simulink model "controladorLEAD"  (R2024b)
settings: Solver=VariableStepAuto  StartTime=0.0  StopTime=50  RelTol=1e-3
values from neighbouring files (symbols this model uses):
  planta = obterPlanta()    [obterMalhaAngular.m]    (also in obterMalhaTangencial.m; simularBarra.m; simularRampa.m)
  saturacoes = obterSaturacao()    [simularBarra.m]    (also in simularRampa.m = obterValoresSaturacao())
  x0 = [Mp_req, t_req]    [ajustarRequisitosEstabilidade.m]
undefined symbols (not defined in the file or in its folder): controlador, theta0
libraries: simulink x1
settings Model: Creator=josal  LastModifiedBy=quantks

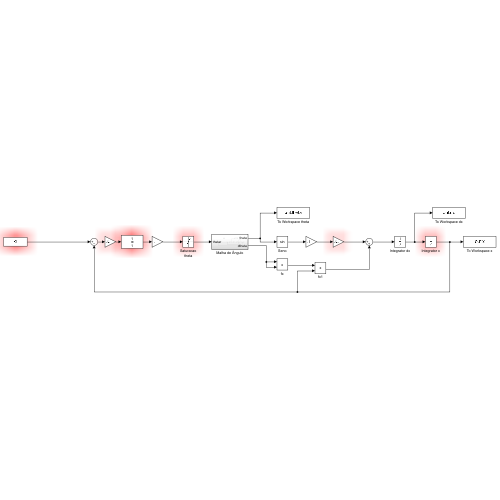
[thumbnail: Simulink's stored preview of the top-level diagram]
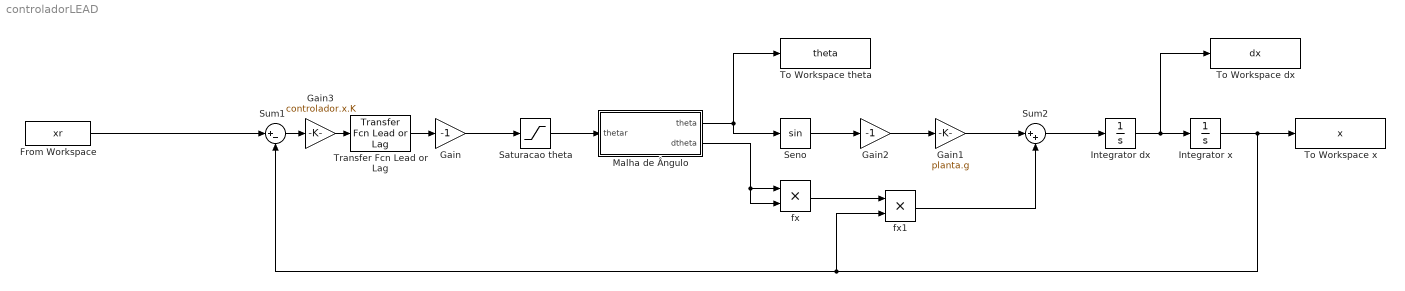
== system controladorLEAD ==
  From Workspace : FromWorkspace  VariableName=xr
  Gain : Gain  Gain=-1
  Gain1 : Gain  Gain=planta.g
  Gain2 : Gain  Gain=-1
  Gain3 : Gain  Gain=controlador.x.K
  Integrator dx : Integrator
  Integrator x : Integrator  InitialCondition=x0
  Malha de Ângulo : Subsystem
  Saturacao theta : Saturate  UpperLimit=saturacoes.sat_theta  LowerLimit=-saturacoes.sat_theta
  Seno : Trigonometry
  Sum1 : Sum  Inputs=|+-
  Sum2 : Sum  Inputs=|++
  To Workspace dx : ToWorkspace  VariableName=dx  SaveFormat=Structure With Time  SampleTime=-1
  To Workspace theta : ToWorkspace  VariableName=theta  SaveFormat=Structure With Time  SampleTime=-1
  To Workspace x : ToWorkspace  VariableName=x  SaveFormat=Structure With Time  SampleTime=-1
  Transfer Fcn Lead or Lag : simulink/Discrete/Transfer Fcn Lead or Lag  PoleZ=-1/(controlador.x.alpha*controlador.x.T)  ZeroZ=-1/(controlador.x.T)  ICPrevOutput=0.0  ICPrevInput=0.0  DoSatur=off
  fx : Product
  fx1 : Product
  wires:
  From Workspace/1 -> Sum1/1
  Integrator dx/1 -> To Workspace dx/1, Integrator x/1
  Integrator x/1 -> To Workspace x/1, fx1/2, Sum1/2
  Transfer Fcn Lead or Lag/1 -> Gain/1
  Malha de Ângulo/1(theta) -> Seno/1, To Workspace theta/1
  Seno/1 -> Gain2/1
  Gain2/1 -> Gain1/1
  Malha de Ângulo/2(dtheta) -> fx/2, fx/1
  fx/1 -> fx1/1
  Gain1/1 -> Sum2/1
  Sum2/1 -> Integrator dx/1
  Gain/1 -> Saturacao theta/1
  Saturacao theta/1 -> Malha de Ângulo/1(thetar)
  fx1/1 -> Sum2/2
  Sum1/1 -> Gain3/1
  Gain3/1 -> Transfer Fcn Lead or Lag/1

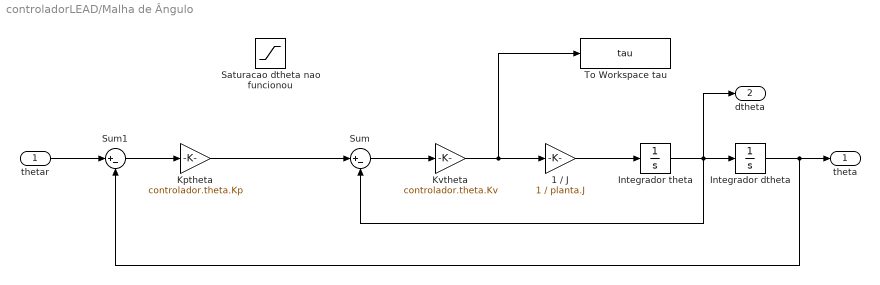
== system controladorLEAD/Malha de Ângulo ==
  thetar : Inport
  1 / J : Gain  Gain=1 / planta.J
  Integrador dtheta : Integrator
  Integrador theta : Integrator  InitialCondition=theta0
  Kptheta : Gain  Gain=controlador.theta.Kp
  Kvtheta : Gain  Gain=controlador.theta.Kv
  Saturacao dtheta nao funcionou : Saturate  UpperLimit=saturacoes.sat_dtheta  LowerLimit=-saturacoes.sat_dtheta
  Sum : Sum  Inputs=|+-
  Sum1 : Sum  Inputs=|+-
  To Workspace tau : ToWorkspace  VariableName=tau  SaveFormat=Structure With Time  SampleTime=-1
  theta : Outport
  dtheta : Outport  Port=2
  wires:
  Integrador theta/1 -> dtheta/1, Sum/2, Integrador dtheta/1
  Sum1/1 -> Kptheta/1
  Integrador dtheta/1 -> Sum1/2, theta/1
  Kvtheta/1 -> 1 / J/1, To Workspace tau/1
  thetar/1 -> Sum1/1
  1 / J/1 -> Integrador theta/1
  Sum/1 -> Kvtheta/1
  Kptheta/1 -> Sum/1
